simulink model "GMCLIB_DecouplingPMSM_BAM_F32"  (Simulink 7.3)
settings: Solver=ode45  StartTime=0.0  StopTime=10.0  RelTol=1e-3
undefined symbols (not defined in the file): f32Kd, f32Kq, s16KdShift, s16KqShift
settings Model: Creator=B17364  LastModifiedBy=B17364

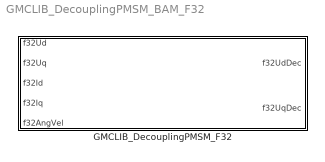
== system GMCLIB_DecouplingPMSM_BAM_F32 ==
  GMCLIB_DecouplingPMSM_F32 : Subsystem  mask(GMCLIB_DecouplingPMSM_F32){f32Kd=f32Kd, s16KdShift=s16KdShift, f32Kq=f32Kq, s16KqShift=s16KqShift}
      mask help: Bit accurate model of decoupling for PMSM model.
      mask init:
      | pos = get_param(gcb, 'Position');width = pos(3) - pos(1); height = pos(4) - pos(2);tX=width/2;tY=height*0.9;
      mask Display: color('black');port_label('input',1,'f32Ud');port_label('input',2,'f32Uq');port_label('input',3,'f32Id');port_label('input',4,'f32Iq');port_label('input',5,'f32AngVel');port_label('output',1,'f32UdDec');port_label('output',2,'f32UqDec');color('black');disp('GMCLIB_DecouplingPMSM_F32');color('blue');text(tX,tY, 'BAM', 'horizontalAlignment', 'center');

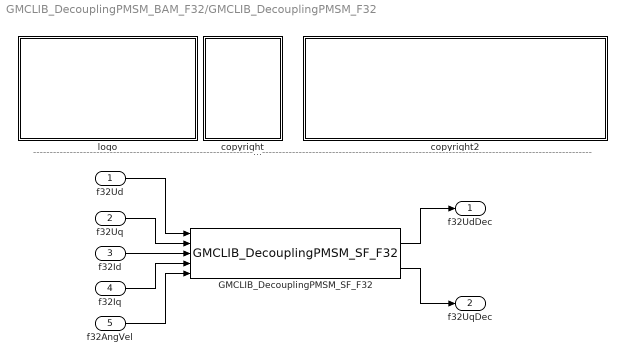
== system GMCLIB_DecouplingPMSM_BAM_F32/GMCLIB_DecouplingPMSM_F32 ==
  note: ---------------------------------------------------------------------------------------------------------------------------------------------------------------------------------------------------
  f32Ud : Inport  OutDataType=fixdt(1, 16)  OutScaling=2^0
  f32Uq : Inport  Port=2  OutDataType=fixdt(1, 16)  OutScaling=2^0
  f32Id : Inport  Port=3  OutDataType=fixdt(1, 16)  OutScaling=2^0
  f32Iq : Inport  Port=4  OutDataType=fixdt(1, 16)  OutScaling=2^0
  f32AngVel : Inport  Port=5  OutDataType=fixdt(1, 16)  OutScaling=2^0
  GMCLIB_DecouplingPMSM_SF_F32 : S-Function  FunctionName=GMCLIB_DecouplingPMSM_SF_F32  Parameters=f32Kd,s16KdShift,f32Kq,s16KqShift  EnableBusSupport=off
  copyright : Subsystem
      mask Display: text(10,90,'FILE:');text(10,75,'DESRIPTION:')text(10,60,'COPYRIGHT:')text(10,45,'VERSION:')text(10,30,'DATE:')
  copyright2 : Subsystem
      mask Display: text(10,90,'GMCLIB_DecouplingPMSM_BAM_F32.mdl');text(10,75,'Decoupling of d and q axis of PMSM model.');text(10,60,'Freescale')text(10,45,'0.1');text(10,30,'14-Sep-2011');
  logo : Subsystem
      mask Display: image(imread('logo.jpg'))
  f32UdDec : Outport  OutDataType=fixdt(1, 16)  OutScaling=2^0
  f32UqDec : Outport  Port=2  OutDataType=fixdt(1, 16)  OutScaling=2^0
  wires:
  f32Ud/1 -> GMCLIB_DecouplingPMSM_SF_F32/1
  f32Uq/1 -> GMCLIB_DecouplingPMSM_SF_F32/2
  f32Id/1 -> GMCLIB_DecouplingPMSM_SF_F32/3
  f32Iq/1 -> GMCLIB_DecouplingPMSM_SF_F32/4
  f32AngVel/1 -> GMCLIB_DecouplingPMSM_SF_F32/5
  GMCLIB_DecouplingPMSM_SF_F32/1 -> f32UdDec/1
  GMCLIB_DecouplingPMSM_SF_F32/2 -> f32UqDec/1

== system GMCLIB_DecouplingPMSM_BAM_F32/GMCLIB_DecouplingPMSM_F32/copyright ==

== system GMCLIB_DecouplingPMSM_BAM_F32/GMCLIB_DecouplingPMSM_F32/copyright2 ==

== system GMCLIB_DecouplingPMSM_BAM_F32/GMCLIB_DecouplingPMSM_F32/logo ==
